simulink model "a3_4_cosine_trigonometry_single_scope"  (R2018a)
settings: Solver=VariableStepAuto  StartTime=0.0  StopTime=10.0  RelTol=1e-3
settings Model: Creator=r0x6f736f646f  LastModifiedBy=r0x6f736f646f

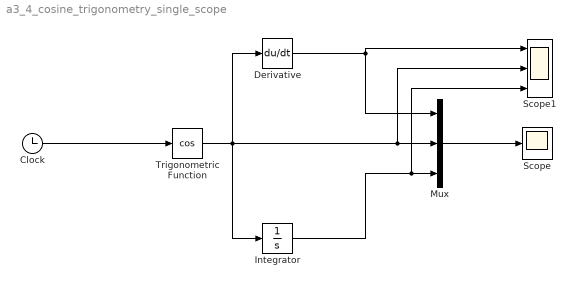
== system a3_4_cosine_trigonometry_single_scope ==
  Clock : Clock
  Derivative : Derivative
  Integrator : Integrator
  Mux : Mux  Inputs=3
  Scope : Scope
  Scope1 : Scope  NumInputPorts=3
  Trigonometric Function : Trigonometry  Operator=cos
  wires:
  Clock/1 -> Trigonometric Function/1
  Trigonometric Function/1 -> Scope1/2, Mux/2, Integrator/1, Derivative/1
  Mux/1 -> Scope/1
  Derivative/1 -> Scope1/1, Mux/1
  Integrator/1 -> Scope1/3, Mux/3
